simulink model "Validacion_simulink_T"  (R2018a)
settings: Solver=VariableStepAuto  StartTime=0.0  StopTime=35  MaxStep=0.005  RelTol=1e-3
values from neighbouring files (symbols this model uses):
  Area = h*w    (= 5e-08)    [Constantes.m]
  cos_theta = (h/(h+w)*cos(theta_plast))+(w/(h+w)*cos(theta_vidrio))    [Constantes.m]
  gamma = sigma*2*(h+w)/(h*w)    (= 1344)    [Constantes.m]
  kappa = 12/(h^2)*(1/(1-(0.63*h/w)))    (= 4956117707.8)    [Constantes.m]
  L1 = 30E-3    (= 0.03)    [Constantes.m]
  L2 = 50E-3    (= 0.05)    [Constantes.m]
  L3 = 70E-3    (= 0.07)    [Constantes.m]
  mu_g = 20*10^-8    (= 2e-07)    [Constantes.m]
  mu_l = 1.13*10^-3    (= 0.00113)    [Constantes.m]
libraries: simulink x2
settings Model: Creator=Pedro  LastModifiedBy=Pedro
settings SolverCC: MaxConsecutiveMinStep=2  ZeroCrossAlgorithm=Adaptive  DecoupledContinuousIntegration=on
settings DebuggingCC: MaxConsecutiveZCsMsg=none  MaskedZcDiagnostic=none  IgnoredZcDiagnostic=none

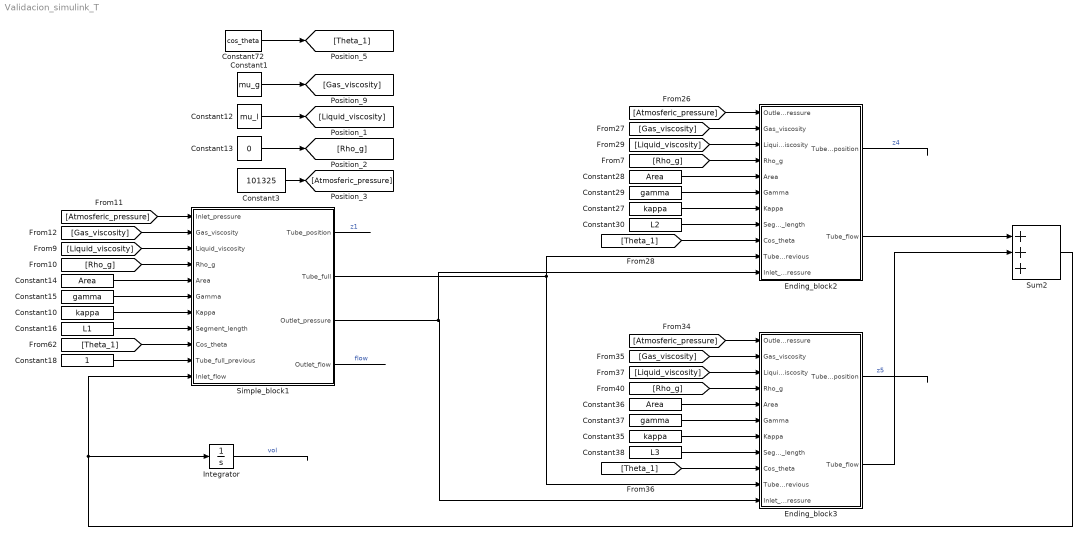
== system Validacion_simulink_T ==
  Constant1 : Constant  Value=mu_g
  Constant10 : Constant  Value=kappa
  Constant12 : Constant  Value=mu_l
  Constant13 : Constant  Value=0
  Constant14 : Constant  Value=Area
  Constant15 : Constant  Value=gamma
  Constant16 : Constant  Value=L1
  Constant18 : Constant
  Constant27 : Constant  Value=kappa
  Constant28 : Constant  Value=Area
  Constant29 : Constant  Value=gamma
  Constant3 : Constant  Value=101325
  Constant30 : Constant  Value=L2  VectorParams1D=off
  Constant35 : Constant  Value=kappa
  Constant36 : Constant  Value=Area
  Constant37 : Constant  Value=gamma
  Constant38 : Constant  Value=L3
  Constant72 : Constant  Value=cos_theta
  Ending_block2 : Subsystem
  Ending_block3 : Subsystem
  Integrator : Integrator
  Simple_block1 : Subsystem
  Sum2 : Sum  Inputs=+++
  wires:
  Constant1/1 -> [Gas_viscosity]
  Constant12/1 -> [Liquid_viscosity]
  Constant13/1 -> [Rho_g]
  Constant3/1 -> [Atmosferic_pressure]
  [Atmosferic_pressure] -> Simple_block1/1(Inlet_pressure)
  [Rho_g] -> Simple_block1/4(Rho_g)
  [Liquid_viscosity] -> Simple_block1/3(Liquid_viscosity)
  [Gas_viscosity] -> Simple_block1/2(Gas_viscosity)
  Constant15/1 -> Simple_block1/6(Gamma)
  Constant14/1 -> Simple_block1/5(Area)
  Constant16/1 -> Simple_block1/8(Segment_length)
  Constant10/1 -> Simple_block1/7(Kappa)
  [Theta_1] -> Simple_block1/9(Cos_theta)
  Constant18/1 -> Simple_block1/10(Tube_full_previous)
  Constant72/1 -> [Theta_1]
  Simple_block1/1(Tube_position) -> ?  "z1"
  Simple_block1/2(Tube_full) -> Ending_block3/10(Tube_full_previous), Ending_block2/10(Tube_full_previous)
  Simple_block1/4(Outlet_flow) -> ?  "flow"
  Ending_block2/2(Tube_flow) -> Sum2/1
  [Rho_g] -> Ending_block2/4(Rho_g)
  [Liquid_viscosity] -> Ending_block2/3(Liquid_viscosity)
  Constant28/1 -> Ending_block2/5(Area)
  Constant27/1 -> Ending_block2/7(Kappa)
  Constant29/1 -> Ending_block2/6(Gamma)
  [Gas_viscosity] -> Ending_block2/2(Gas_viscosity)
  [Atmosferic_pressure] -> Ending_block2/1(Outlet_pressure)
  [Theta_1] -> Ending_block2/9(Cos_theta)
  Constant30/1 -> Ending_block2/8(Segment_length)
  Ending_block2/1(Tube_position) -> ?  "z4"
  [Atmosferic_pressure] -> Ending_block3/1(Outlet_pressure)
  Constant38/1 -> Ending_block3/8(Segment_length)
  Constant35/1 -> Ending_block3/7(Kappa)
  [Liquid_viscosity] -> Ending_block3/3(Liquid_viscosity)
  Constant36/1 -> Ending_block3/5(Area)
  [Theta_1] -> Ending_block3/9(Cos_theta)
  [Rho_g] -> Ending_block3/4(Rho_g)
  Constant37/1 -> Ending_block3/6(Gamma)
  [Gas_viscosity] -> Ending_block3/2(Gas_viscosity)
  Ending_block3/1(Tube_position) -> ?  "z5"
  Ending_block3/2(Tube_flow) -> Sum2/2
  Sum2/1 -> Integrator/1, Simple_block1/11(Inlet_flow)
  Simple_block1/3(Outlet_pressure) -> Ending_block2/11(Inlet_pressure), Ending_block3/11(Inlet_pressure)
  Integrator/1 -> ?  "vol"

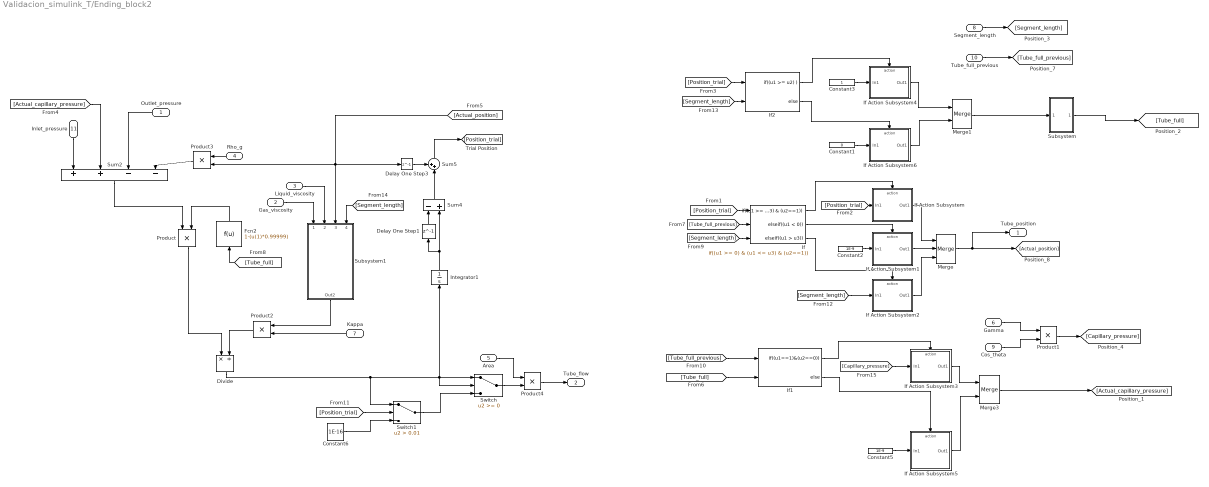
== system Validacion_simulink_T/Ending_block2 ==
  Outlet_pressure : Inport
  Gas_viscosity : Inport  Port=2
  Liquid_viscosity : Inport  Port=3
  Rho_g : Inport  Port=4
  Area : Inport  Port=5
  Gamma : Inport  Port=6
  Kappa : Inport  Port=7
  Segment_length : Inport  Port=8
  Cos_theta : Inport  Port=9
  Tube_full_previous : Inport  Port=10
  Inlet_pressure : Inport  Port=11
  Constant1 : Constant  Value=0
  Constant2 : Constant  Value=1E-9
  Constant3 : Constant
  Constant5 : Constant  Value=1E-9
  Constant6 : Constant  Value=1E-16
  Delay One Step1 : Delay  DelayLength=1
  Delay One Step3 : Delay  DelayLength=1
  Divide : Product  Inputs=*/
  Fcn2 : Fcn  Expr=1-(u(1)*0.99999)
  If : If  NumInputs=3  IfExpression=(u1 >= 0) & (u1 <= u3) & (u2==1)  ElseIfExpressions=(u1 < 0),(u1 > u3)  ShowElse=off
  If Action Subsystem : Subsystem  TreatAsAtomicUnit=on
  If Action Subsystem1 : Subsystem  TreatAsAtomicUnit=on
  If Action Subsystem2 : Subsystem  TreatAsAtomicUnit=on
  If Action Subsystem3 : Subsystem  TreatAsAtomicUnit=on
  If Action Subsystem4 : Subsystem  TreatAsAtomicUnit=on
  If Action Subsystem5 : Subsystem  TreatAsAtomicUnit=on
  If Action Subsystem6 : Subsystem  TreatAsAtomicUnit=on
  If1 : If  NumInputs=2  IfExpression=(u1==1)&(u2==0)
  If2 : If  NumInputs=2  IfExpression=(u1 >= u2)
  Integrator1 : Integrator
  Merge : Merge  Inputs=3
  Merge1 : Merge
  Merge3 : Merge
  Product{,1..4} (5 alike) : Product
  Subsystem : Subsystem
  Subsystem1 : Subsystem
  Sum2 : Sum  Inputs=++--
  Sum4 : Sum  Inputs=-+
  Sum5 : Sum  Inputs=++|
  Switch : Switch
  Switch1 : Switch  Criteria=u2 > Threshold  Threshold=0.01
  Tube_position : Outport
  Tube_flow : Outport  Port=2
  wires:
  Delay One Step1/1 -> Sum4/1
  Integrator1/1 -> Delay One Step1/1, Sum4/2
  Sum5/1 -> [Position_trial]
  Delay One Step3/1 -> Sum5/1
  Inlet_pressure/1 -> Sum2/1
  Outlet_pressure/1 -> Sum2/3
  [Position_trial] -> If Action Subsystem/1(In1)
  If Action Subsystem/1(Out1) -> Merge/1
  If/1 -> If Action Subsystem/Action
  [Actual_capillary_pressure] -> Sum2/2
  [Position_trial] -> If/1
  Sum4/1 -> Sum5/2
  Constant2/1 -> If Action Subsystem1/1(In1)
  If Action Subsystem1/1(Out1) -> Merge/2
  If/2 -> If Action Subsystem1/Action
  Tube_full_previous/1 -> [Tube_full_previous]
  [Tube_full_previous] -> If/2
  If Action Subsystem2/1(Out1) -> Merge/3
  [Segment_length] -> If/3
  If/3 -> If Action Subsystem2/Action
  Merge/1 -> Tube_position/1, [Actual_position]
  If1/2 -> If Action Subsystem5/Action
  If1/1 -> If Action Subsystem3/Action
  If Action Subsystem3/1(Out1) -> Merge3/1
  Constant5/1 -> If Action Subsystem5/1(In1)
  If Action Subsystem5/1(Out1) -> Merge3/2
  [Tube_full_previous] -> If1/1
  [Position_trial] -> If2/1
  Constant1/1 -> If Action Subsystem6/1(In1)
  If2/1 -> If Action Subsystem4/Action
  If Action Subsystem6/1(Out1) -> Merge1/2
  If Action Subsystem4/1(Out1) -> Merge1/1
  If2/2 -> If Action Subsystem6/Action
  Constant3/1 -> If Action Subsystem4/1(In1)
  [Actual_position] -> Subsystem1/3(Actual_position), Delay One Step3/1, Product3/2
  [Tube_full] -> If1/2
  [Tube_full] -> Fcn2/1
  Sum2/1 -> Product/1
  Product/1 -> Divide/1
  Divide/1 -> Switch1/1, Integrator1/1, Switch/1, Switch/2
  Switch1/1 -> Switch/3
  Constant6/1 -> Switch1/3
  [Position_trial] -> Switch1/2
  Merge3/1 -> [Actual_capillary_pressure]
  Fcn2/1 -> Product/2
  Merge1/1 -> Subsystem/1(In1)
  Subsystem/1(Out1) -> [Tube_full]
  Product3/1 -> Sum2/4
  Gas_viscosity/1 -> Subsystem1/1(Gas_viscosity)
  Liquid_viscosity/1 -> Subsystem1/2(Liquid_viscosity1)
  Segment_length/1 -> [Segment_length]
  [Segment_length] -> If Action Subsystem2/1(In1)
  [Segment_length] -> If2/2
  [Segment_length] -> Subsystem1/4(Segment_length)
  Gamma/1 -> Product1/1
  Cos_theta/1 -> Product1/2
  Product1/1 -> [Capillary_pressure]
  [Capillary_pressure] -> If Action Subsystem3/1(In1)
  Product2/1 -> Divide/2
  Subsystem1/1(Out2) -> Product2/1
  Kappa/1 -> Product2/2
  Rho_g/1 -> Product3/1
  Switch/1 -> Product4/2
  Product4/1 -> Tube_flow/1
  Area/1 -> Product4/1

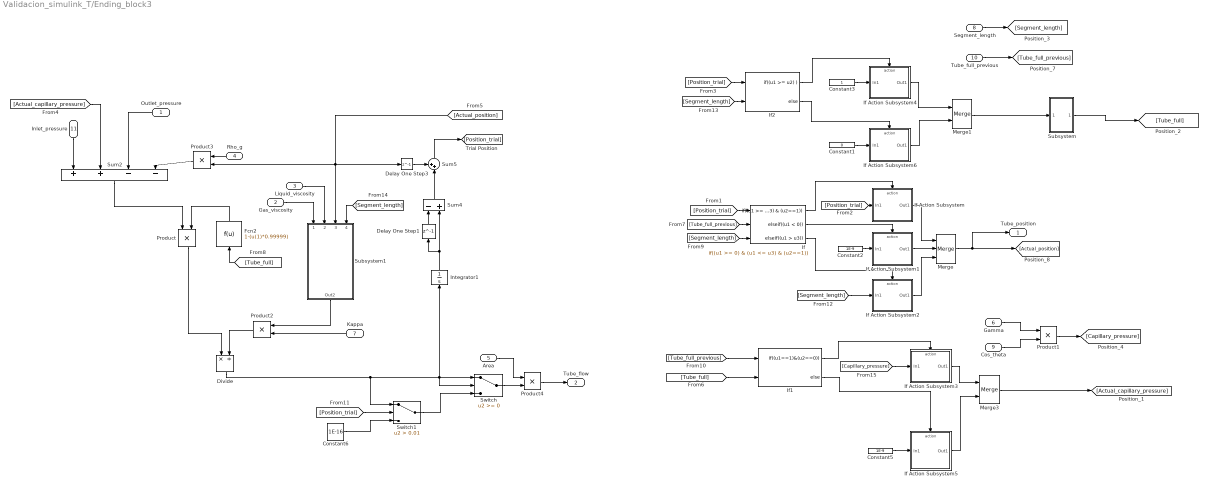
== system Validacion_simulink_T/Ending_block3 ==
  Outlet_pressure : Inport
  Gas_viscosity : Inport  Port=2
  Liquid_viscosity : Inport  Port=3
  Rho_g : Inport  Port=4
  Area : Inport  Port=5
  Gamma : Inport  Port=6
  Kappa : Inport  Port=7
  Segment_length : Inport  Port=8
  Cos_theta : Inport  Port=9
  Tube_full_previous : Inport  Port=10
  Inlet_pressure : Inport  Port=11
  Constant1 : Constant  Value=0
  Constant2 : Constant  Value=1E-9
  Constant3 : Constant
  Constant5 : Constant  Value=1E-9
  Constant6 : Constant  Value=1E-16
  Delay One Step1 : Delay  DelayLength=1
  Delay One Step3 : Delay  DelayLength=1
  Divide : Product  Inputs=*/
  Fcn2 : Fcn  Expr=1-(u(1)*0.99999)
  If : If  NumInputs=3  IfExpression=(u1 >= 0) & (u1 <= u3) & (u2==1)  ElseIfExpressions=(u1 < 0),(u1 > u3)  ShowElse=off
  If Action Subsystem : Subsystem  TreatAsAtomicUnit=on
  If Action Subsystem1 : Subsystem  TreatAsAtomicUnit=on
  If Action Subsystem2 : Subsystem  TreatAsAtomicUnit=on
  If Action Subsystem3 : Subsystem  TreatAsAtomicUnit=on
  If Action Subsystem4 : Subsystem  TreatAsAtomicUnit=on
  If Action Subsystem5 : Subsystem  TreatAsAtomicUnit=on
  If Action Subsystem6 : Subsystem  TreatAsAtomicUnit=on
  If1 : If  NumInputs=2  IfExpression=(u1==1)&(u2==0)
  If2 : If  NumInputs=2  IfExpression=(u1 >= u2)
  Integrator1 : Integrator
  Merge : Merge  Inputs=3
  Merge1 : Merge
  Merge3 : Merge
  Product{,1..4} (5 alike) : Product
  Subsystem : Subsystem
  Subsystem1 : Subsystem
  Sum2 : Sum  Inputs=++--
  Sum4 : Sum  Inputs=-+
  Sum5 : Sum  Inputs=++|
  Switch : Switch
  Switch1 : Switch  Criteria=u2 > Threshold  Threshold=0.01
  Tube_position : Outport
  Tube_flow : Outport  Port=2
  wires:
  Delay One Step1/1 -> Sum4/1
  Integrator1/1 -> Delay One Step1/1, Sum4/2
  Sum5/1 -> [Position_trial]
  Delay One Step3/1 -> Sum5/1
  Inlet_pressure/1 -> Sum2/1
  Outlet_pressure/1 -> Sum2/3
  [Position_trial] -> If Action Subsystem/1(In1)
  If Action Subsystem/1(Out1) -> Merge/1
  If/1 -> If Action Subsystem/Action
  [Actual_capillary_pressure] -> Sum2/2
  [Position_trial] -> If/1
  Sum4/1 -> Sum5/2
  Constant2/1 -> If Action Subsystem1/1(In1)
  If Action Subsystem1/1(Out1) -> Merge/2
  If/2 -> If Action Subsystem1/Action
  Tube_full_previous/1 -> [Tube_full_previous]
  [Tube_full_previous] -> If/2
  If Action Subsystem2/1(Out1) -> Merge/3
  [Segment_length] -> If/3
  If/3 -> If Action Subsystem2/Action
  Merge/1 -> Tube_position/1, [Actual_position]
  If1/2 -> If Action Subsystem5/Action
  If1/1 -> If Action Subsystem3/Action
  If Action Subsystem3/1(Out1) -> Merge3/1
  Constant5/1 -> If Action Subsystem5/1(In1)
  If Action Subsystem5/1(Out1) -> Merge3/2
  [Tube_full_previous] -> If1/1
  [Position_trial] -> If2/1
  Constant1/1 -> If Action Subsystem6/1(In1)
  If2/1 -> If Action Subsystem4/Action
  If Action Subsystem6/1(Out1) -> Merge1/2
  If Action Subsystem4/1(Out1) -> Merge1/1
  If2/2 -> If Action Subsystem6/Action
  Constant3/1 -> If Action Subsystem4/1(In1)
  [Actual_position] -> Subsystem1/3(Actual_position), Delay One Step3/1, Product3/2
  [Tube_full] -> If1/2
  [Tube_full] -> Fcn2/1
  Sum2/1 -> Product/1
  Product/1 -> Divide/1
  Divide/1 -> Switch1/1, Integrator1/1, Switch/1, Switch/2
  Switch1/1 -> Switch/3
  Constant6/1 -> Switch1/3
  [Position_trial] -> Switch1/2
  Merge3/1 -> [Actual_capillary_pressure]
  Fcn2/1 -> Product/2
  Merge1/1 -> Subsystem/1(In1)
  Subsystem/1(Out1) -> [Tube_full]
  Product3/1 -> Sum2/4
  Gas_viscosity/1 -> Subsystem1/1(Gas_viscosity)
  Liquid_viscosity/1 -> Subsystem1/2(Liquid_viscosity1)
  Segment_length/1 -> [Segment_length]
  [Segment_length] -> If Action Subsystem2/1(In1)
  [Segment_length] -> If2/2
  [Segment_length] -> Subsystem1/4(Segment_length)
  Gamma/1 -> Product1/1
  Cos_theta/1 -> Product1/2
  Product1/1 -> [Capillary_pressure]
  [Capillary_pressure] -> If Action Subsystem3/1(In1)
  Product2/1 -> Divide/2
  Subsystem1/1(Out2) -> Product2/1
  Kappa/1 -> Product2/2
  Rho_g/1 -> Product3/1
  Switch/1 -> Product4/2
  Product4/1 -> Tube_flow/1
  Area/1 -> Product4/1

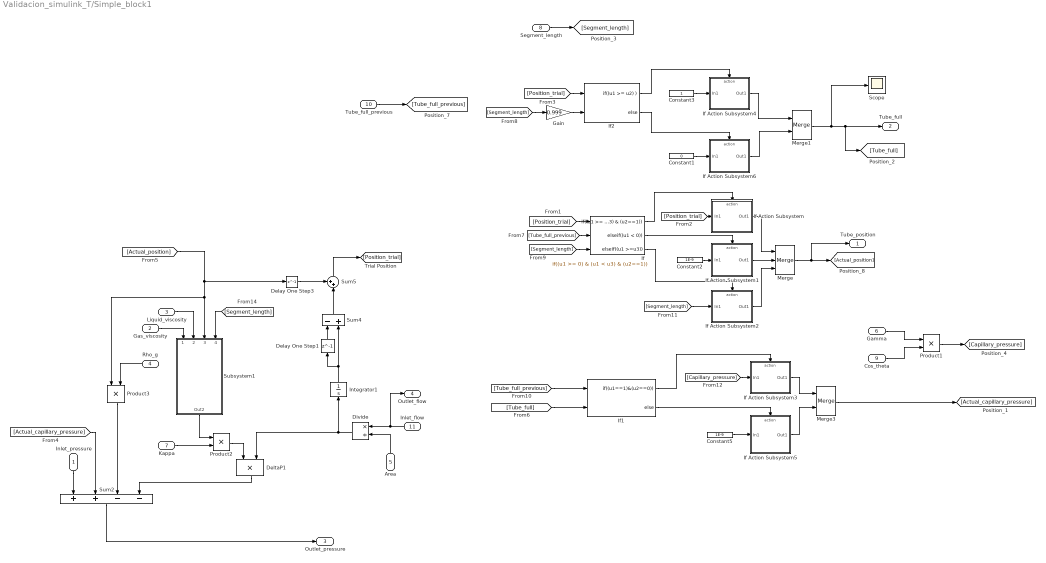
== system Validacion_simulink_T/Simple_block1 ==
  Inlet_pressure : Inport
  Gas_viscosity : Inport  Port=2
  Liquid_viscosity : Inport  Port=3
  Rho_g : Inport  Port=4
  Area : Inport  Port=5
  Gamma : Inport  Port=6
  Kappa : Inport  Port=7
  Segment_length : Inport  Port=8
  Cos_theta : Inport  Port=9
  Tube_full_previous : Inport  Port=10
  Inlet_flow : Inport  Port=11
  Constant1 : Constant  Value=0
  Constant2 : Constant  Value=1E-9
  Constant3 : Constant
  Constant5 : Constant  Value=1E-9
  Delay One Step1 : Delay  DelayLength=1
  Delay One Step3 : Delay  DelayLength=1
  DeltaP1 : Product  Inputs=**
  Divide : Product  Inputs=*/
  Gain : Gain  Gain=0.999
  If : If  NumInputs=3  IfExpression=(u1 >= 0) & (u1 < u3) & (u2==1)  ElseIfExpressions=(u1 < 0),(u1 >=u3)  ShowElse=off
  If Action Subsystem : Subsystem  TreatAsAtomicUnit=on
  If Action Subsystem1 : Subsystem  TreatAsAtomicUnit=on
  If Action Subsystem2 : Subsystem  TreatAsAtomicUnit=on
  If Action Subsystem3 : Subsystem  TreatAsAtomicUnit=on
  If Action Subsystem4 : Subsystem  TreatAsAtomicUnit=on
  If Action Subsystem5 : Subsystem  TreatAsAtomicUnit=on
  If Action Subsystem6 : Subsystem  TreatAsAtomicUnit=on
  If1 : If  NumInputs=2  IfExpression=(u1==1)&(u2==0)
  If2 : If  NumInputs=2  IfExpression=(u1 >= u2)
  Integrator1 : Integrator  InitialCondition=0.001
  Merge : Merge  Inputs=3
  Merge1 : Merge
  Merge3 : Merge
  Product1 : Product
  Product2 : Product
  Product3 : Product
  Scope : Scope
  Subsystem1 : Subsystem
  Sum2 : Sum  Inputs=++--
  Sum4 : Sum  Inputs=-+
  Sum5 : Sum  Inputs=++|
  Tube_position : Outport
  Tube_full : Outport  Port=2
  Outlet_pressure : Outport  Port=3
  Outlet_flow : Outport  Port=4
  wires:
  Delay One Step1/1 -> Sum4/1
  Integrator1/1 -> Delay One Step1/1, Sum4/2
  Sum5/1 -> [Position_trial]
  Delay One Step3/1 -> Sum5/1
  Inlet_pressure/1 -> Sum2/1
  [Position_trial] -> If Action Subsystem/1(In1)
  If Action Subsystem/1(Out1) -> Merge/1
  If/1 -> If Action Subsystem/Action
  [Actual_capillary_pressure] -> Sum2/2
  [Position_trial] -> If/1
  Sum4/1 -> Sum5/2
  Constant2/1 -> If Action Subsystem1/1(In1)
  If Action Subsystem1/1(Out1) -> Merge/2
  If/2 -> If Action Subsystem1/Action
  Tube_full_previous/1 -> [Tube_full_previous]
  [Tube_full_previous] -> If/2
  If Action Subsystem2/1(Out1) -> Merge/3
  [Segment_length] -> If Action Subsystem2/1(In1)
  If/3 -> If Action Subsystem2/Action
  Merge/1 -> Tube_position/1, [Actual_position]
  [Capillary_pressure] -> If Action Subsystem3/1(In1)
  If1/2 -> If Action Subsystem5/Action
  If1/1 -> If Action Subsystem3/Action
  If Action Subsystem3/1(Out1) -> Merge3/1
  Constant5/1 -> If Action Subsystem5/1(In1)
  If Action Subsystem5/1(Out1) -> Merge3/2
  [Tube_full_previous] -> If1/1
  [Position_trial] -> If2/1
  Constant1/1 -> If Action Subsystem6/1(In1)
  If2/1 -> If Action Subsystem4/Action
  If Action Subsystem6/1(Out1) -> Merge1/2
  If Action Subsystem4/1(Out1) -> Merge1/1
  If2/2 -> If Action Subsystem6/Action
  Constant3/1 -> If Action Subsystem4/1(In1)
  Inlet_flow/1 -> Divide/1, Outlet_flow/1
  [Tube_full] -> If1/2
  Sum2/1 -> Outlet_pressure/1
  Merge1/1 -> Scope/1, [Tube_full], Tube_full/1
  Merge3/1 -> [Actual_capillary_pressure]
  DeltaP1/1 -> Sum2/4
  Segment_length/1 -> [Segment_length]
  [Segment_length] -> Gain/1
  [Segment_length] -> If/3
  [Segment_length] -> Subsystem1/4(Segment_length)
  Gas_viscosity/1 -> Subsystem1/1(Gas_viscosity)
  [Actual_position] -> Product3/1, Subsystem1/3(Actual_position), Delay One Step3/1
  Liquid_viscosity/1 -> Subsystem1/2(Liquid_viscosity1)
  Rho_g/1 -> Product3/2
  Product3/1 -> Sum2/3
  Divide/1 -> DeltaP1/2, Integrator1/1
  Area/1 -> Divide/2
  Product1/1 -> [Capillary_pressure]
  Gamma/1 -> Product1/1
  Product2/1 -> DeltaP1/1
  Subsystem1/1(Out2) -> Product2/1
  Kappa/1 -> Product2/2
  Gain/1 -> If2/2
  Cos_theta/1 -> Product1/2

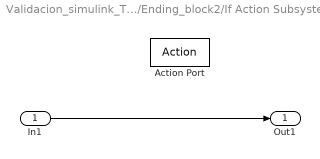
== system Validacion_simulink_T/Ending_block2/If Action Subsystem ==
  In1 : Inport
  Action Port : ActionPort  ActionType=then
  Out1 : Outport
  wires:
  In1/1 -> Out1/1

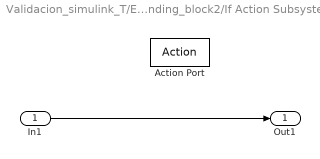
== system Validacion_simulink_T/Ending_block2/If Action Subsystem1 ==
  In1 : Inport
  Action Port : ActionPort  ActionType=elseif
  Out1 : Outport
  wires:
  In1/1 -> Out1/1

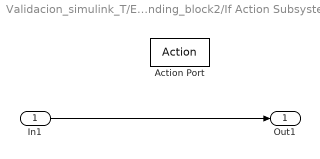
== system Validacion_simulink_T/Ending_block2/If Action Subsystem2 ==
  In1 : Inport
  Action Port : ActionPort  ActionType=elseif
  Out1 : Outport
  wires:
  In1/1 -> Out1/1

== system Validacion_simulink_T/Ending_block2/If Action Subsystem3 ==
  In1 : Inport
  Action Port : ActionPort  ActionType=then
  Out1 : Outport
  wires:
  In1/1 -> Out1/1

== system Validacion_simulink_T/Ending_block2/If Action Subsystem4 ==
  In1 : Inport
  Action Port : ActionPort  ActionType=then
  Out1 : Outport
  wires:
  In1/1 -> Out1/1

== system Validacion_simulink_T/Ending_block2/If Action Subsystem5 ==
  In1 : Inport
  Action Port : ActionPort  ActionType=else
  Out1 : Outport
  wires:
  In1/1 -> Out1/1

== system Validacion_simulink_T/Ending_block2/If Action Subsystem6 ==
  In1 : Inport
  Action Port : ActionPort  ActionType=else
  Out1 : Outport
  wires:
  In1/1 -> Out1/1

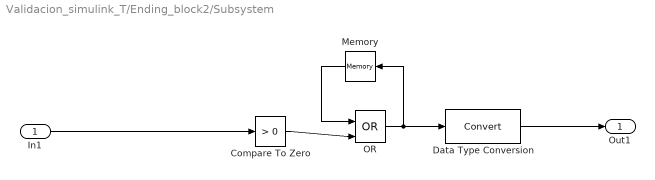
== system Validacion_simulink_T/Ending_block2/Subsystem ==
  In1 : Inport
  Compare To Zero : simulink/Logic and Bit Operations/Compare To Zero  relop=>  OutDataTypeStr=boolean
  Data Type Conversion : DataTypeConversion
  Memory : Memory
  OR : Logic  Operator=OR  IconShape=distinctive  AllPortsSameDT=off  OutDataTypeStr=boolean
  Out1 : Outport
  wires:
  In1/1 -> Compare To Zero/1
  OR/1 -> Memory/1, Data Type Conversion/1
  Compare To Zero/1 -> OR/2
  Data Type Conversion/1 -> Out1/1
  Memory/1 -> OR/1

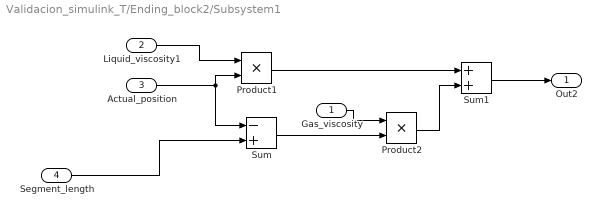
== system Validacion_simulink_T/Ending_block2/Subsystem1 ==
  Gas_viscosity : Inport
  Liquid_viscosity1 : Inport  Port=2
  Actual_position : Inport  Port=3
  Segment_length : Inport  Port=4
  Product1 : Product
  Product2 : Product
  Sum : Sum  Inputs=-+
  Sum1 : Sum
  Out2 : Outport
  wires:
  Liquid_viscosity1/1 -> Product1/1
  Sum/1 -> Product2/2
  Actual_position/1 -> Product1/2, Sum/1
  Product2/1 -> Sum1/2
  Product1/1 -> Sum1/1
  Segment_length/1 -> Sum/2
  Gas_viscosity/1 -> Product2/1
  Sum1/1 -> Out2/1

== system Validacion_simulink_T/Ending_block3/If Action Subsystem ==
  In1 : Inport
  Action Port : ActionPort  ActionType=then
  Out1 : Outport
  wires:
  In1/1 -> Out1/1

== system Validacion_simulink_T/Ending_block3/If Action Subsystem1 ==
  In1 : Inport
  Action Port : ActionPort  ActionType=elseif
  Out1 : Outport
  wires:
  In1/1 -> Out1/1

== system Validacion_simulink_T/Ending_block3/If Action Subsystem2 ==
  In1 : Inport
  Action Port : ActionPort  ActionType=elseif
  Out1 : Outport
  wires:
  In1/1 -> Out1/1

== system Validacion_simulink_T/Ending_block3/If Action Subsystem3 ==
  In1 : Inport
  Action Port : ActionPort  ActionType=then
  Out1 : Outport
  wires:
  In1/1 -> Out1/1

== system Validacion_simulink_T/Ending_block3/If Action Subsystem4 ==
  In1 : Inport
  Action Port : ActionPort  ActionType=then
  Out1 : Outport
  wires:
  In1/1 -> Out1/1

== system Validacion_simulink_T/Ending_block3/If Action Subsystem5 ==
  In1 : Inport
  Action Port : ActionPort  ActionType=else
  Out1 : Outport
  wires:
  In1/1 -> Out1/1

== system Validacion_simulink_T/Ending_block3/If Action Subsystem6 ==
  In1 : Inport
  Action Port : ActionPort  ActionType=else
  Out1 : Outport
  wires:
  In1/1 -> Out1/1

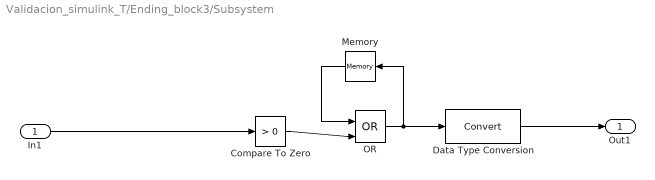
== system Validacion_simulink_T/Ending_block3/Subsystem ==
  In1 : Inport
  Compare To Zero : simulink/Logic and Bit Operations/Compare To Zero  relop=>  OutDataTypeStr=boolean
  Data Type Conversion : DataTypeConversion
  Memory : Memory
  OR : Logic  Operator=OR  IconShape=distinctive  AllPortsSameDT=off  OutDataTypeStr=boolean
  Out1 : Outport
  wires:
  In1/1 -> Compare To Zero/1
  OR/1 -> Memory/1, Data Type Conversion/1
  Compare To Zero/1 -> OR/2
  Data Type Conversion/1 -> Out1/1
  Memory/1 -> OR/1

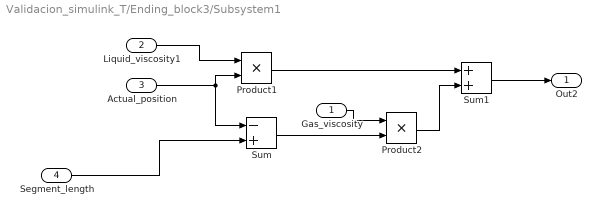
== system Validacion_simulink_T/Ending_block3/Subsystem1 ==
  Gas_viscosity : Inport
  Liquid_viscosity1 : Inport  Port=2
  Actual_position : Inport  Port=3
  Segment_length : Inport  Port=4
  Product1 : Product
  Product2 : Product
  Sum : Sum  Inputs=-+
  Sum1 : Sum
  Out2 : Outport
  wires:
  Liquid_viscosity1/1 -> Product1/1
  Sum/1 -> Product2/2
  Actual_position/1 -> Product1/2, Sum/1
  Product2/1 -> Sum1/2
  Product1/1 -> Sum1/1
  Segment_length/1 -> Sum/2
  Gas_viscosity/1 -> Product2/1
  Sum1/1 -> Out2/1

== system Validacion_simulink_T/Simple_block1/If Action Subsystem ==
  In1 : Inport
  Action Port : ActionPort  ActionType=then
  Out1 : Outport
  wires:
  In1/1 -> Out1/1

== system Validacion_simulink_T/Simple_block1/If Action Subsystem1 ==
  In1 : Inport
  Action Port : ActionPort  ActionType=elseif
  Out1 : Outport
  wires:
  In1/1 -> Out1/1

== system Validacion_simulink_T/Simple_block1/If Action Subsystem2 ==
  In1 : Inport
  Action Port : ActionPort  ActionType=elseif
  Out1 : Outport
  wires:
  In1/1 -> Out1/1

== system Validacion_simulink_T/Simple_block1/If Action Subsystem3 ==
  In1 : Inport
  Action Port : ActionPort  ActionType=then
  Out1 : Outport
  wires:
  In1/1 -> Out1/1

== system Validacion_simulink_T/Simple_block1/If Action Subsystem4 ==
  In1 : Inport
  Action Port : ActionPort  ActionType=then
  Out1 : Outport
  wires:
  In1/1 -> Out1/1

== system Validacion_simulink_T/Simple_block1/If Action Subsystem5 ==
  In1 : Inport
  Action Port : ActionPort  ActionType=else
  Out1 : Outport
  wires:
  In1/1 -> Out1/1

== system Validacion_simulink_T/Simple_block1/If Action Subsystem6 ==
  In1 : Inport
  Action Port : ActionPort  ActionType=else
  Out1 : Outport
  wires:
  In1/1 -> Out1/1

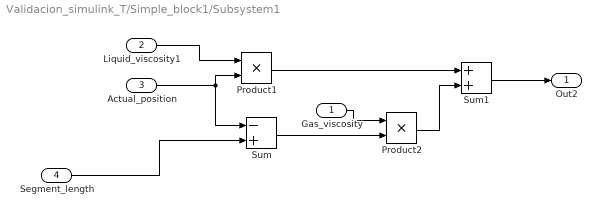
== system Validacion_simulink_T/Simple_block1/Subsystem1 ==
  Gas_viscosity : Inport
  Liquid_viscosity1 : Inport  Port=2
  Actual_position : Inport  Port=3
  Segment_length : Inport  Port=4
  Product1 : Product
  Product2 : Product
  Sum : Sum  Inputs=-+
  Sum1 : Sum
  Out2 : Outport
  wires:
  Liquid_viscosity1/1 -> Product1/1
  Sum/1 -> Product2/2
  Actual_position/1 -> Product1/2, Sum/1
  Product2/1 -> Sum1/2
  Product1/1 -> Sum1/1
  Segment_length/1 -> Sum/2
  Gas_viscosity/1 -> Product2/1
  Sum1/1 -> Out2/1
